simulink model "debugmotor"  (R2024a)
settings: Solver=VariableStepAuto  StartTime=0.0  StopTime=10  RelTol=1e-3
InitFcn:
  | stm32_pmsm_foc_data
undefined symbols (not defined in the file): PWM_frequency, target
libraries: mcbcontrolslib x7, simulink x2, slpidlib x2, mcbsensorlessestimatorlib x1, mcbplantlib x1, autolibpmsmexterior x1
settings Model: Creator=wsl  LastModifiedBy=wsl
settings DebuggingCC: ParameterPrecisionLossMsg=none

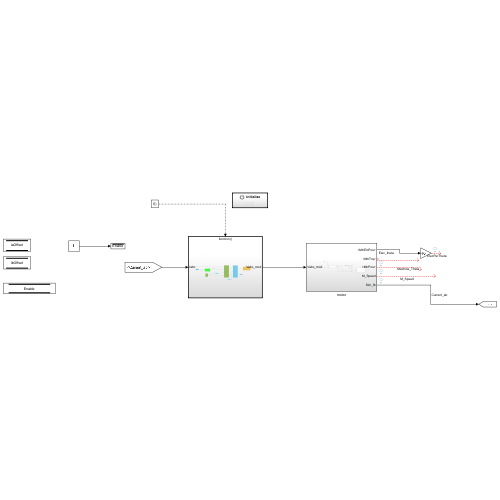
[thumbnail: Simulink's stored preview of the top-level diagram]
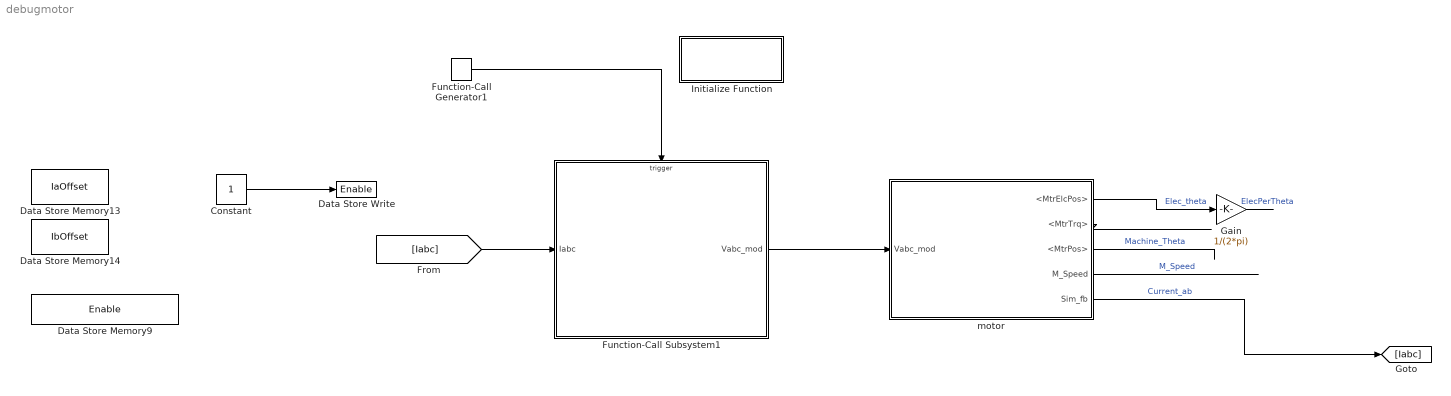
== system debugmotor ==
  Constant : Constant
  Data Store Memory13 : DataStoreMemory  DataStoreName=IaOffset  WriteAfterWriteMsg=warning  ShowAdditionalParam=off
  Data Store Memory14 : DataStoreMemory  DataStoreName=IbOffset  WriteAfterWriteMsg=warning  ShowAdditionalParam=off
  Data Store Memory9 : DataStoreMemory  DataStoreName=Enable  WriteAfterWriteMsg=warning  ShowAdditionalParam=off
  Data Store Write : DataStoreWrite  DataStoreName=Enable  IndexOptions=Index vector (dialog)  Indices=1  OutputSizes=1
  Function-Call Generator1 : simulink/Ports & Subsystems/Function-Call Generator  sample_time=Ts  numberOfIterations=1  DisallowWideOutput=off
  Function-Call Subsystem1 : Subsystem  TreatAsAtomicUnit=on
  Gain : Gain  Gain=1/(2*pi)
  Initialize Function : Subsystem  TreatAsAtomicUnit=on
  motor : Subsystem
  wires:
  motor/3(<MtrPos>) -> ?  "Machine_Theta"
  motor/5(Sim_fb) -> [Iabc]  "Current_ab"
  motor/2(<MtrTrq>) -> ?
  motor/4(M_Speed) -> ?  "M_Speed"
  Function-Call Generator1/1 -> Function-Call Subsystem1/Trigger
  Function-Call Subsystem1/1(Vabc_mod) -> motor/1(Vabc_mod)
  [Iabc] -> Function-Call Subsystem1/1(Iabc)
  Constant/1 -> Data Store Write/1
  motor/1(<MtrElcPos>) -> Gain/1  "Elec_theta"
  Gain/1 -> ?  "ElecPerTheta"

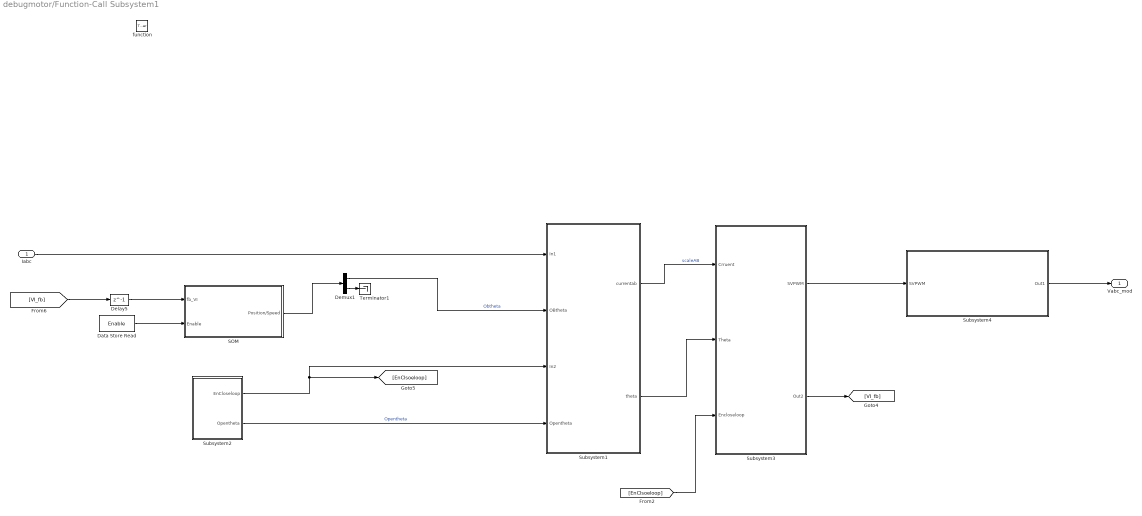
== system debugmotor/Function-Call Subsystem1 ==
  Iabc : Inport
  function : TriggerPort  TriggerType=function-call  VariantControl=(inherit)
  Data Store Read : DataStoreRead  DataStoreName=Enable  IndexOptions=Index vector (dialog)  Indices=1  OutputSizes=1
  Delay5 : Delay  DelayLength=1
  Demux1 : Demux  Outputs=2
  SOM : Subsystem
  Subsystem1 : Subsystem
  Subsystem2 : Subsystem
  Subsystem3 : Subsystem
  Subsystem4 : Subsystem
  Terminator1 : Terminator
  Vabc_mod : Outport
  wires:
  Subsystem1/1(currentab) -> Subsystem3/1(Crruent)  "scaleAB"
  Subsystem2/1(EnCloseloop) -> [EnClsoeloop], Subsystem1/3(In2)
  Subsystem2/2(Opentheta) -> Subsystem1/4(Opentheta)  "Opentheta"
  Demux1/2 -> Terminator1/1
  SOM/1(Position/Speed) -> Demux1/1
  Delay5/1 -> SOM/1(fb_VI)
  Data Store Read/1 -> SOM/2(Enable)
  [VI_fb] -> Delay5/1
  Demux1/1 -> Subsystem1/2(OBtheta)  "Obtheta"
  Iabc/1 -> Subsystem1/1(In1)
  Subsystem1/2(theta) -> Subsystem3/2(Theta)
  Subsystem3/2(Out2) -> [VI_fb]
  Subsystem3/1(SVPWM) -> Subsystem4/1(SVPWM)
  Subsystem4/1(Out1) -> Vabc_mod/1
  [EnClsoeloop] -> Subsystem3/3(Encloseloop)

== system debugmotor/Initialize Function ==
  Data Store Write : DataStoreWrite  DataStoreName=IaOffset  IndexOptions=Index vector (dialog)  Indices=1  OutputSizes=1
  Data Store Write1 : DataStoreWrite  DataStoreName=IbOffset  IndexOptions=Index vector (dialog)  Indices=1  OutputSizes=1
  Event Listener : EventListener  DisableCoverage=on  EventName=reset
  Testing get offset : Constant  Value=2075  OutDataTypeStr=int16
  Testing get offset1 : Constant  Value=2051  OutDataTypeStr=int16
  wires:
  Testing get offset1/1 -> Data Store Write/1
  Testing get offset/1 -> Data Store Write1/1

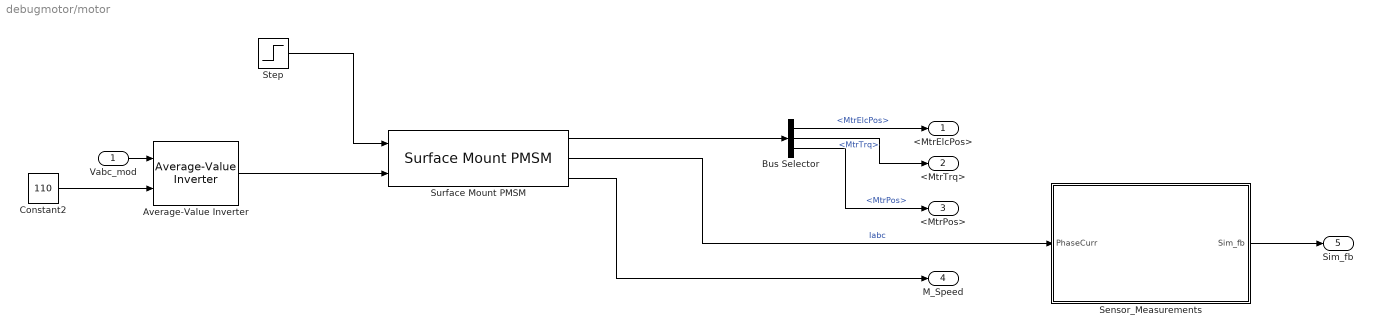
== system debugmotor/motor ==
  Vabc_mod : Inport
  Average-Value Inverter : mcbplantlib/Average-Value Inverter
  Bus Selector : BusSelector  OutputSignals=MtrElcPos,MtrTrq,MtrPos
  Constant2 : Constant  Value=110
  Sensor_Measurements : Subsystem
  Step : Step  After=0.15  SampleTime=0.01
  Surface Mount PMSM : autolibpmsmexterior/Surface Mount PMSM  port_config=Torque  sim_type=Discrete  Ts=5e-6  P=2  Rs=18.0  Ldq_=0.0407  KConstText=Back-emf constant (Ke):  lambda_pm=0.2205  Ke=29  Kt=1.323  mechanical=[0.0027, 4.924e-4, 0.05]  idq0=[0 0]  theta_init=0  omega_init=0  KConst=0.2205  lambda_pm_calc=0.079943  RefBlkName='autolibpmsmexterior/Surface Mount PMSM'  aMode=5  Ldq="[0.0017      0.0017]"
  <MtrElcPos> : Outport
  <MtrTrq> : Outport  Port=2
  <MtrPos> : Outport  Port=3
  M_Speed : Outport  Port=4
  Sim_fb : Outport  Port=5
  wires:
  Surface Mount PMSM/3 -> M_Speed/1
  Constant2/1 -> Average-Value Inverter/2
  Vabc_mod/1 -> Average-Value Inverter/1
  Average-Value Inverter/1 -> Surface Mount PMSM/2
  Step/1 -> Surface Mount PMSM/1
  Surface Mount PMSM/2 -> Sensor_Measurements/1(PhaseCurr)  "Iabc"
  Surface Mount PMSM/1 -> Bus Selector/1
  Bus Selector/1 -> <MtrElcPos>/1  "<MtrElcPos>"
  Bus Selector/2 -> <MtrTrq>/1  "<MtrTrq>"
  Bus Selector/3 -> <MtrPos>/1  "<MtrPos>"
  Sensor_Measurements/1(Sim_fb) -> Sim_fb/1

== system debugmotor/Function-Call Subsystem1/SOM ==
  fb_VI : Inport
  Enable : Inport  Port=2
  Demux1 : Demux
  Logical Operator : Logic  Operator=NOT  IconShape=distinctive  AllPortsSameDT=off  OutDataTypeStr=boolean
  Mux : Mux  Inputs=2
  Sliding Mode Observer : mcbsensorlessestimatorlib/Sliding Mode Observer  InputUnit=Per-unit  BlkSampleTime=50e-6  StatorResistance=18.1  StatorInductance=0.0407  MaxApplicationSpeed=2500  PolePairs=2  MaxStatorVoltage=110/1.732  MaxStatorCurrent=1  DisturbanceObserverGain=0.9  CurrentObserverGain=0.004938  CutoffFreq=500  PositionUnit=Per unit  PositionDataType=single  SpeedUnit=RPM  PerUnitSpeed=PU_System.N_base  SpeedDataType=single
  Position/Speed : Outport
  wires:
  Logical Operator/1 -> Sliding Mode Observer/5
  Mux/1 -> Position/Speed/1
  Demux1/3 -> Sliding Mode Observer/3  "Ialpha"
  fb_VI/1 -> Demux1/1
  Sliding Mode Observer/2 -> Mux/2
  Demux1/2 -> Sliding Mode Observer/2
  Sliding Mode Observer/1 -> Mux/1
  Enable/1 -> Logical Operator/1
  Demux1/1 -> Sliding Mode Observer/1
  Demux1/4 -> Sliding Mode Observer/4  "Ibeta"

== system debugmotor/Function-Call Subsystem1/Subsystem1 ==
  In1 : Inport
  OBtheta : Inport  Port=2
  In2 : Inport  Port=3
  Opentheta : Inport  Port=4
  Feedbackt_Current : Subsystem
  Switch : Switch  Criteria=u2 ~= 0  Threshold=0.1  SaturateOnIntegerOverflow=off  InputSameDT=off
  currentab : Outport
  theta : Outport  Port=2
  wires:
  Opentheta/1 -> Switch/3  "Eps"
  In2/1 -> Switch/2
  Switch/1 -> theta/1
  OBtheta/1 -> Switch/1
  In1/1 -> Feedbackt_Current/1(In1)
  Feedbackt_Current/1(currentab) -> currentab/1

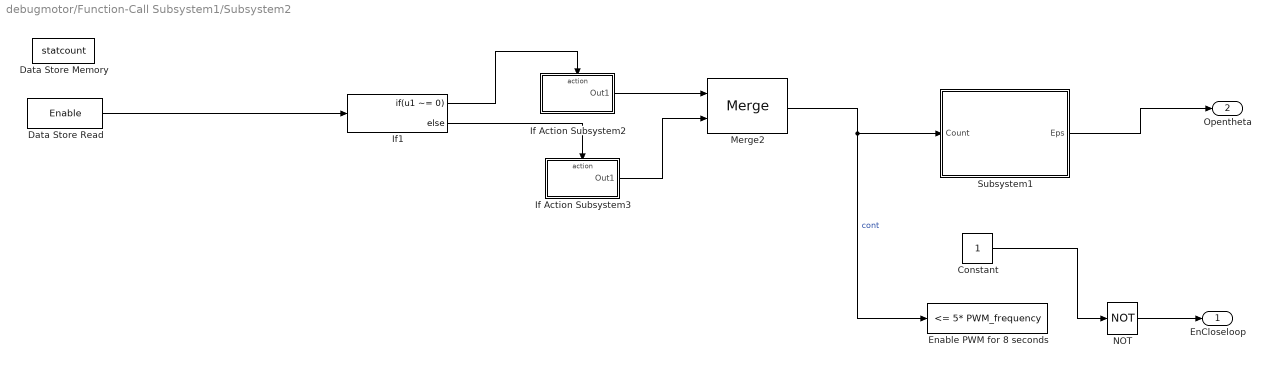
== system debugmotor/Function-Call Subsystem1/Subsystem2 ==
  Constant : Constant
  Data Store Memory : DataStoreMemory  DataStoreName=statcount  WriteAfterWriteMsg=warning  ShowAdditionalParam=off
  Data Store Read : DataStoreRead  DataStoreName=Enable  IndexOptions=Index vector (dialog)  Indices=1  OutputSizes=1
  Enable PWM for 8 seconds : simulink/Logic and Bit Operations/Compare To Constant  relop=<=  const=5* PWM_frequency  OutDataTypeStr=boolean
  If Action Subsystem2 : Subsystem  TreatAsAtomicUnit=on
  If Action Subsystem3 : Subsystem  TreatAsAtomicUnit=on
  If1 : If  IfExpression=u1 ~= 0
  Merge2 : Merge
  NOT : Logic  Operator=NOT  IconShape=distinctive  AllPortsSameDT=off  OutDataTypeStr=boolean
  Subsystem1 : Subsystem
  EnCloseloop : Outport  OutputWhenDisabled=reset  InitialOutput=0  VectorParamsAs1DForOutWhenUnconnected=off
  Opentheta : Outport  Port=2
  wires:
  If1/2 -> If Action Subsystem3/Action
  If1/1 -> If Action Subsystem2/Action
  If Action Subsystem3/1(Out1) -> Merge2/2
  If Action Subsystem2/1(Out1) -> Merge2/1
  Merge2/1 -> Enable PWM for 8 seconds/1, Subsystem1/1(Count)  "cont"
  Data Store Read/1 -> If1/1
  NOT/1 -> EnCloseloop/1
  Subsystem1/1(Eps) -> Opentheta/1
  Constant/1 -> NOT/1

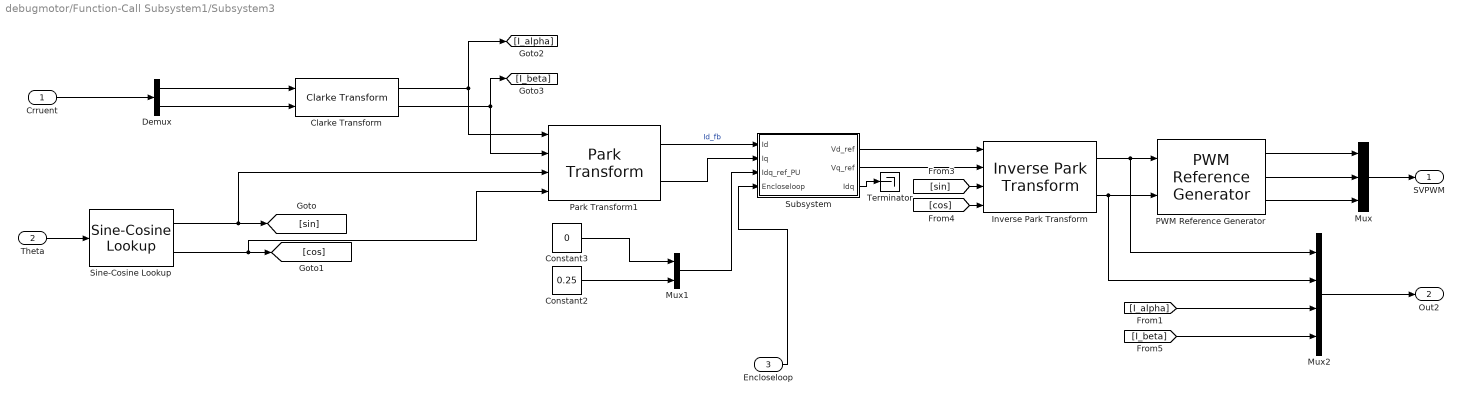
== system debugmotor/Function-Call Subsystem1/Subsystem3 ==
  Crruent : Inport
  Theta : Inport  Port=2
  Encloseloop : Inport  Port=3
  Clarke Transform : mcbcontrolslib/Clarke Transform  VariantControl=Variant2  PhaseInput=Two inputs  EnPowerInv=off
      settings: LibrarySourceBlock=mcbhdllib/Controls/Math Transforms/Clarke Transform
  Constant2 : Constant  Value=0.25  OutDataTypeStr=single
  Constant3 : Constant  Value=0  OutDataTypeStr=single
  Demux : Demux  Outputs=2
  Inverse Park Transform : mcbcontrolslib/Inverse Park Transform  PhaseInput=Two inputs  AxisAlignment=D-axis  ThetaInput=Sine and Cosine electrical position  AngleInput=Per-unit  N_points=1024
  Mux : Mux  Inputs=3
  Mux1 : Mux  Inputs=2
  Mux2 : Mux
  PWM Reference Generator : mcbcontrolslib/PWM Reference Generator  inSignal=Valphabeta  modType=SVM: space vector modulation
      settings: LibrarySourceBlock=mcblib/Controls/Math Transforms/PWM Reference Generator
  Park Transform1 : mcbcontrolslib/Park Transform  PhaseInput=Two inputs  AxisAlignment=D-axis  ThetaInput=Sine and Cosine electrical position  AngleInput=Per-unit  N_points=1024
      settings: LibrarySourceBlock=mcbhdllib/Controls/Math Transforms/Park Transform
  Sine-Cosine Lookup : mcbcontrolslib/Sine-Cosine Lookup  AngleInput=Per-unit  N_points=1024  DatatypeInput=Inherit from input  Datatype=single
  Subsystem : Subsystem
  Terminator : Terminator
  SVPWM : Outport
  Out2 : Outport  Port=2
  wires:
  Constant2/1 -> Mux1/2
  PWM Reference Generator/2 -> Mux/2
  Park Transform1/2 -> Subsystem/2(Iq)
  [cos] -> Inverse Park Transform/4
  Demux/2 -> Clarke Transform/2
  Sine-Cosine Lookup/1 -> Park Transform1/3, [sin]
  Subsystem/3(Idq) -> Terminator/1
  Demux/1 -> Clarke Transform/1
  Inverse Park Transform/1 -> Mux2/1, PWM Reference Generator/1
  Sine-Cosine Lookup/2 -> Park Transform1/4, [cos]
  Mux/1 -> SVPWM/1
  PWM Reference Generator/1 -> Mux/1
  Constant3/1 -> Mux1/1
  [sin] -> Inverse Park Transform/3
  Inverse Park Transform/2 -> Mux2/2, PWM Reference Generator/2
  [I_alpha] -> Mux2/3
  Clarke Transform/2 -> Park Transform1/2, [I_beta]
  Clarke Transform/1 -> Park Transform1/1, [I_alpha]
  Park Transform1/1 -> Subsystem/1(Id)  "Id_fb"
  [I_beta] -> Mux2/4
  Encloseloop/1 -> Subsystem/4(Encloseloop)
  Crruent/1 -> Demux/1
  PWM Reference Generator/3 -> Mux/3
  Subsystem/2(Vq_ref) -> Inverse Park Transform/2
  Mux1/1 -> Subsystem/3(Idq_ref_PU)
  Subsystem/1(Vd_ref) -> Inverse Park Transform/1
  Mux2/1 -> Out2/1
  Theta/1 -> Sine-Cosine Lookup/1

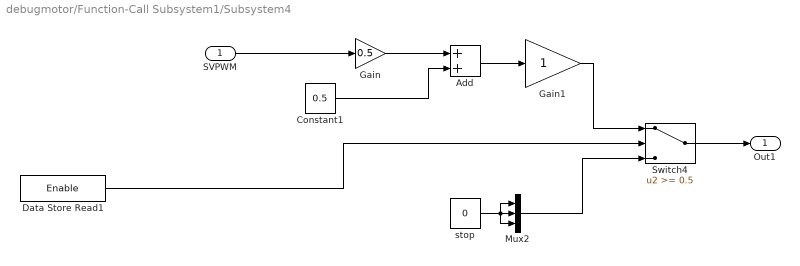
== system debugmotor/Function-Call Subsystem1/Subsystem4 ==
  SVPWM : Inport
  Add : Sum
  Constant1 : Constant  Value=0.5  OutDataTypeStr=single
  Data Store Read1 : DataStoreRead  DataStoreName=Enable  IndexOptions=Index vector (dialog)  Indices=1  OutputSizes=1
  Gain : Gain  Gain=0.5  OutDataTypeStr=single  RndMeth=Simplest
  Gain1 : Gain  OutDataTypeStr=single
  Mux2 : Mux  Inputs=3
  Switch4 : Switch  Threshold=0.5  SaturateOnIntegerOverflow=off  InputSameDT=off
  stop : Constant  Value=0  OutDataTypeStr=uint16
  Out1 : Outport
  wires:
  Gain1/1 -> Switch4/1
  Gain/1 -> Add/1
  Add/1 -> Gain1/1
  Data Store Read1/1 -> Switch4/2
  stop/1 -> Mux2/2, Mux2/3, Mux2/1
  Constant1/1 -> Add/2
  SVPWM/1 -> Gain/1
  Mux2/1 -> Switch4/3
  Switch4/1 -> Out1/1

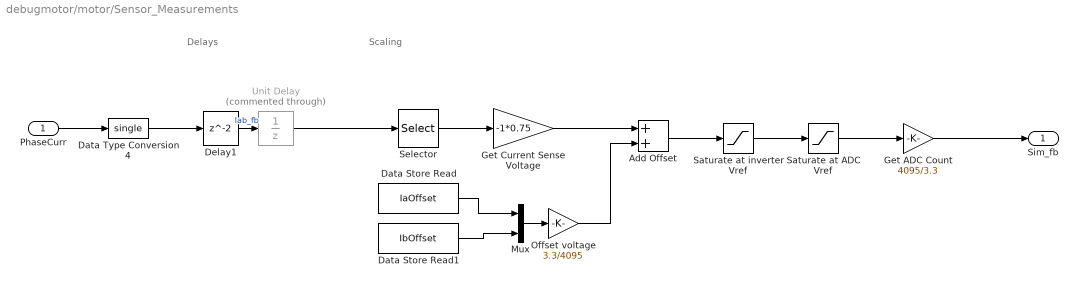
== system debugmotor/motor/Sensor_Measurements ==
  note: Scaling
  note: Delays
  PhaseCurr : Inport
  Add Offset : Sum  RndMeth=Simplest
  Data Store Read : DataStoreRead  DataStoreName=IaOffset  IndexOptions=Index vector (dialog)  Indices=1  OutputSizes=1
  Data Store Read1 : DataStoreRead  DataStoreName=IbOffset  IndexOptions=Index vector (dialog)  Indices=1  OutputSizes=1
  Data Type Conversion4 : DataTypeConversion  OutDataTypeStr=single  RndMeth=Simplest  SaturateOnIntegerOverflow=off
  Delay1 : Delay
  Get ADC Count : Gain  Gain=4095/3.3  OutMin=0  OutMax=target.ADC_MaxCount  OutDataTypeStr=uint16  RndMeth=Simplest
  Get Current Sense Voltage : Gain  Gain=-1*0.75  RndMeth=Simplest  OutDataTypeStr=Inherit: Same as input
  Mux : Mux  Inputs=2
  Offset voltage : Gain  Gain=3.3/4095  RndMeth=Simplest
  Saturate at ADC Vref : Saturate  UpperLimit=3.3  LowerLimit=0
  Saturate at inverter Vref : Saturate  UpperLimit=3.3  LowerLimit=0
  Selector : Selector  InputPortWidth=3  IndexOptions=Index vector (dialog)  Indices=[1 2]  OutputSizes=1
  Unit Delay : UnitDelay  Commented=through  SampleTime=-1  HasFrameUpgradeWarning=on
  Sim_fb : Outport  VectorParamsAs1DForOutWhenUnconnected=off
  wires:
  Delay1/1 -> Unit Delay/1  "Iab_fb"
  Data Type Conversion4/1 -> Delay1/1
  PhaseCurr/1 -> Data Type Conversion4/1
  Get ADC Count/1 -> Sim_fb/1
  Add Offset/1 -> Saturate at inverter Vref/1
  Saturate at inverter Vref/1 -> Saturate at ADC Vref/1
  Get Current Sense Voltage/1 -> Add Offset/1
  Saturate at ADC Vref/1 -> Get ADC Count/1
  Selector/1 -> Get Current Sense Voltage/1
  Offset voltage/1 -> Add Offset/2
  Unit Delay/1 -> Selector/1
  Data Store Read/1 -> Mux/1
  Data Store Read1/1 -> Mux/2
  Mux/1 -> Offset voltage/1

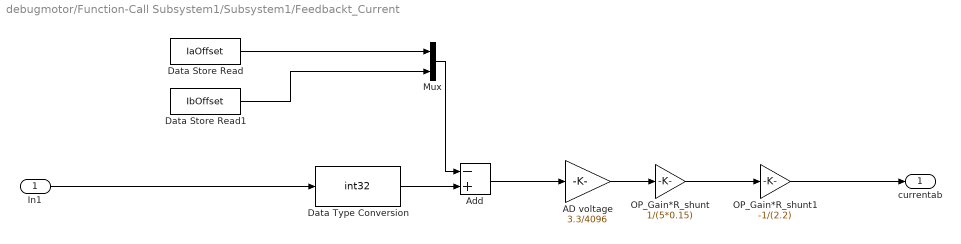
== system debugmotor/Function-Call Subsystem1/Subsystem1/Feedbackt_Current ==
  In1 : Inport
  AD voltage : Gain  Gain=3.3/4096  ParamDataTypeStr=single
  Add : Sum  Inputs=-+
  Data Store Read : DataStoreRead  DataStoreName=IaOffset  IndexOptions=Index vector (dialog)  Indices=1  OutputSizes=1
  Data Store Read1 : DataStoreRead  DataStoreName=IbOffset  IndexOptions=Index vector (dialog)  Indices=1  OutputSizes=1
  Data Type Conversion : DataTypeConversion  OutDataTypeStr=int32  ConvertRealWorld=Stored Integer (SI)  RndMeth=Simplest  SaturateOnIntegerOverflow=off
  Mux : Mux  Inputs=2
  OP_Gain*R_shunt : Gain  Gain=1/(5*0.15)  ParamDataTypeStr=single
  OP_Gain*R_shunt1 : Gain  Gain=-1/(2.2)  ParamDataTypeStr=single
  currentab : Outport
  wires:
  Add/1 -> AD voltage/1
  AD voltage/1 -> OP_Gain*R_shunt/1
  Mux/1 -> Add/1
  Data Type Conversion/1 -> Add/2
  Data Store Read/1 -> Mux/1
  Data Store Read1/1 -> Mux/2
  In1/1 -> Data Type Conversion/1
  OP_Gain*R_shunt1/1 -> currentab/1
  OP_Gain*R_shunt/1 -> OP_Gain*R_shunt1/1

== system debugmotor/Function-Call Subsystem1/Subsystem2/If Action Subsystem2 ==
  Action Port : ActionPort  ActionPortLabel=if(u1 ~= 0)
  Add1 : Sum  SaturateOnIntegerOverflow=on
  Constant : Constant  OutDataTypeStr=uint32
  Data Store Read : DataStoreRead  DataStoreName=statcount  IndexOptions=Index vector (dialog)  Indices=1  OutputSizes=1
  Data Store Write : DataStoreWrite  DataStoreName=statcount  IndexOptions=Index vector (dialog)  Indices=1  OutputSizes=1
  Out1 : Outport
  wires:
  Add1/1 -> Data Store Write/1, Out1/1
  Data Store Read/1 -> Add1/2
  Constant/1 -> Add1/1

== system debugmotor/Function-Call Subsystem1/Subsystem2/If Action Subsystem3 ==
  Action Port : ActionPort  ActionPortLabel=else
  Constant15 : Constant  Value=0  OutDataTypeStr=uint32
  Data Store Write : DataStoreWrite  DataStoreName=statcount  IndexOptions=Index vector (dialog)  Indices=1  OutputSizes=1
  Out1 : Outport
  wires:
  Constant15/1 -> Out1/1, Data Store Write/1

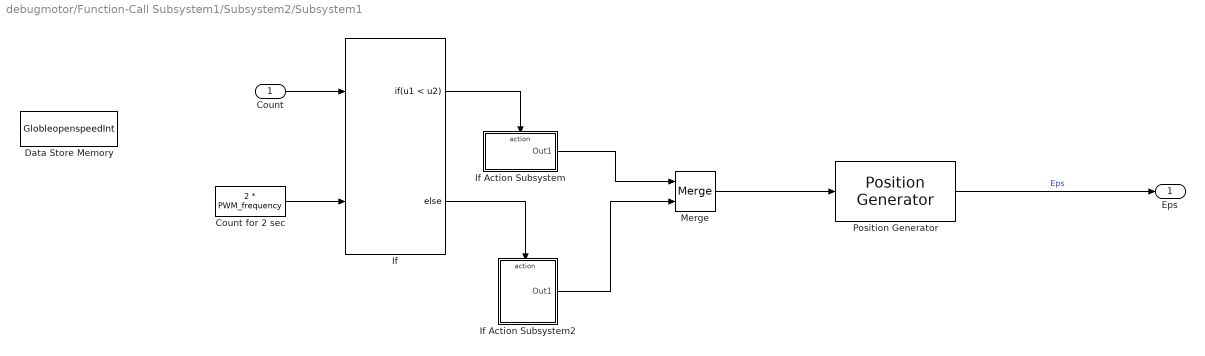
== system debugmotor/Function-Call Subsystem1/Subsystem2/Subsystem1 ==
  Count : Inport
  Count for 2 sec : Constant  Value=2 * PWM_frequency  OutDataTypeStr=uint32  SampleTime=-1
  Data Store Memory : DataStoreMemory  DataStoreName=GlobleopenspeedInt  WriteAfterWriteMsg=warning  ShowAdditionalParam=off
  If : If  NumInputs=2  IfExpression=u1 < u2
  If Action Subsystem : Subsystem  TreatAsAtomicUnit=on
  If Action Subsystem2 : Subsystem  TreatAsAtomicUnit=on
  Merge : Merge
  Position Generator : mcbcontrolslib/Position Generator  AngleOutput=Per-unit  ExternalReset=none  Offset=0
  Eps : Outport
  wires:
  If Action Subsystem/1(Out1) -> Merge/1
  If/1 -> If Action Subsystem/Action
  If Action Subsystem2/1(Out1) -> Merge/2
  Count/1 -> If/1
  If/2 -> If Action Subsystem2/Action
  Count for 2 sec/1 -> If/2
  Merge/1 -> Position Generator/1
  Position Generator/1 -> Eps/1  "Eps"

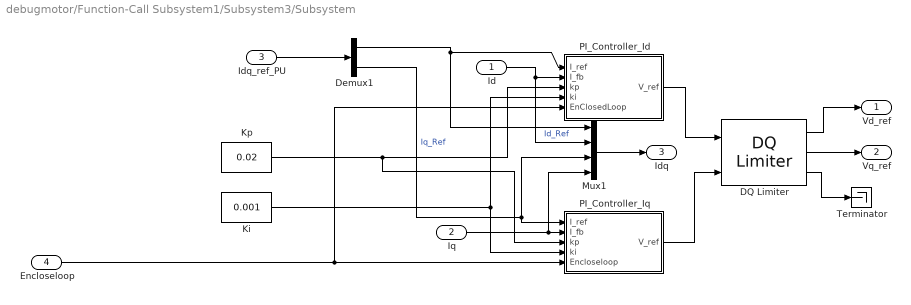
== system debugmotor/Function-Call Subsystem1/Subsystem3/Subsystem ==
  Id : Inport
  Iq : Inport  Port=2
  Idq_ref_PU : Inport  Port=3
  Encloseloop : Inport  Port=4
  DQ Limiter : mcbcontrolslib/DQ Limiter  satMethodInputType=Specify via dialog  satMethodSelected=D-Q equivalence  satLimitInputType=Specify via dialog  Vmax=0.95
  Demux1 : Demux  Outputs=2
  Ki : Constant  Value=0.001  OutDataTypeStr=single  SampleTime=-1
  Kp : Constant  Value=0.02  OutDataTypeStr=single  SampleTime=-1
  Mux1 : Mux
  PI_Controller_Id : Subsystem
  PI_Controller_Iq : Subsystem
  Terminator : Terminator
  Vd_ref : Outport  VectorParamsAs1DForOutWhenUnconnected=off
  Vq_ref : Outport  Port=2  VectorParamsAs1DForOutWhenUnconnected=off
  Idq : Outport  Port=3  VectorParamsAs1DForOutWhenUnconnected=off
  wires:
  DQ Limiter/1 -> Vd_ref/1
  Demux1/2 -> Mux1/3, PI_Controller_Iq/1(I_ref)  "Iq_Ref"
  Id/1 -> Mux1/2, PI_Controller_Id/2(I_fb)
  Demux1/1 -> Mux1/1, PI_Controller_Id/1(I_ref)  "Id_Ref"
  Idq_ref_PU/1 -> Demux1/1
  Iq/1 -> Mux1/4, PI_Controller_Iq/2(I_fb)
  Mux1/1 -> Idq/1
  PI_Controller_Iq/1(V_ref) -> DQ Limiter/2
  DQ Limiter/2 -> Vq_ref/1
  PI_Controller_Id/1(V_ref) -> DQ Limiter/1
  DQ Limiter/3 -> Terminator/1
  Kp/1 -> PI_Controller_Id/3(kp), PI_Controller_Iq/3(kp)
  Ki/1 -> PI_Controller_Iq/4(ki), PI_Controller_Id/4(ki)
  Encloseloop/1 -> PI_Controller_Id/5(EnClosedLoop), PI_Controller_Iq/5(Encloseloop)

== system debugmotor/Function-Call Subsystem1/Subsystem2/Subsystem1/If Action Subsystem ==
  Action Port : ActionPort  ActionPortLabel=if(u1 < u2)
  Constant : Constant  Value=0  OutDataTypeStr=single
  Data Store Write : DataStoreWrite  DataStoreName=GlobleopenspeedInt  IndexOptions=Index vector (dialog)  Indices=1  OutputSizes=1
  Out1 : Outport
  wires:
  Constant/1 -> Out1/1, Data Store Write/1

== system debugmotor/Function-Call Subsystem1/Subsystem2/Subsystem1/If Action Subsystem2 ==
  Action Port : ActionPort  ActionPortLabel=else
  Add1 : Sum
  Constant2 : Constant  Value=50e-6  VectorParams1D=off  OutDataTypeStr=single
  Data Store Read : DataStoreRead  DataStoreName=GlobleopenspeedInt  IndexOptions=Index vector (dialog)  Indices=1  OutputSizes=1
  Data Store Write : DataStoreWrite  DataStoreName=GlobleopenspeedInt  IndexOptions=Index vector (dialog)  Indices=1  OutputSizes=1
  Multiply1 : Gain  Gain=1/PWM_frequency  OutDataTypeStr=Inherit: Same as input
  Saturate to 'motor.calibSpeed' RPM : Saturate  UpperLimit=2 *300/60  LowerLimit=0
  Out1 : Outport
  wires:
  Constant2/1 -> Add1/1
  Saturate to 'motor.calibSpeed' RPM/1 -> Data Store Write/1, Multiply1/1
  Data Store Read/1 -> Add1/2
  Add1/1 -> Saturate to 'motor.calibSpeed' RPM/1
  Multiply1/1 -> Out1/1

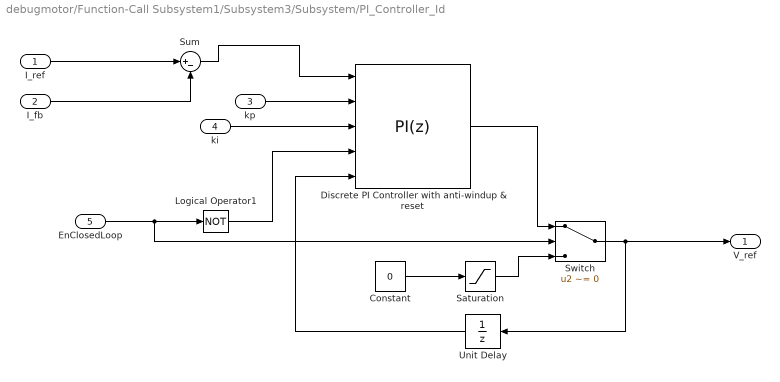
== system debugmotor/Function-Call Subsystem1/Subsystem3/Subsystem/PI_Controller_Id ==
  I_ref : Inport
  I_fb : Inport  Port=2
  kp : Inport  Port=3
  ki : Inport  Port=4
  EnClosedLoop : Inport  Port=5
  Constant : Constant  Value=0
  Discrete PI Controller with anti-windup & reset : slpidlib/PID Controller  Controller=PI  Form=Parallel  TimeDomain=Discrete-time  UseExternalTs=off  SampleTime=-1  IntegratorMethod=Forward Euler  FilterMethod=Forward Euler  ControllerParametersSource=external  P=1  I=1  UseKiTs=on  D=0  UseExternalDerivativeSource=off  N=100  UseFilter=on  TunerSelectOption=Transfer Function Based (PID Tuner App)  InitialConditionSource=external  InitialConditionForIntegrator=0  InitialConditionForFilter=0  DifferentiatorICPrevScaledInput=0  ExternalReset=level  TrackingMode=off  Kt=1  LimitOutput=on  SatLimitsSource=internal  UpperSaturationLimit=1  LowerSaturationLimit=-1  LinearizeAsGain=on  AntiWindupMode=clamping  Kb=1  LimitIntegrator=off  UpperIntegratorSaturationLimit=inf  LowerIntegratorSaturationLimit=-inf  RndMeth=Simplest  POutMin=[]  POutMax=[]  IOutMin=[]  IOutMax=[]  DOutMin=[]  DOutMax=[]  NOutMin=[]  NOutMax=[]  SumOutMin=[]  SumOutMax=[]  SaturationOutDataTypeStr=Inherit: Inherit via back propagation  SaturationOutMin=[]  SaturationOutMax=[]  PParamMin=[]  PParamMax=[]  IParamMin=[]  IParamMax=[]  DParamMin=[]  DParamMax=[]  NParamMin=[]  NParamMax=[]  KbParamMin=[]  KbParamMax=[]  KtParamMin=[]  KtParamMax=[]  KbOutMin=[]  KbOutMax=[]  KtOutMin=[]  KtOutMax=[]  IntegratorOutMin=[]  IntegratorOutMax=[]  FilterOutMin=[]  FilterOutMax=[]  SumI1OutMin=[]  SumI1OutMax=[]  SumI2OutMin=[]  SumI2OutMax=[]  SumI3OutMin=[]  SumI3OutMax=[]  SumI4OutMin=[]  SumI4OutMax=[]  SumDOutMin=[]  SumDOutMax=[]  DifferentiatorOutMin=[]  DifferentiatorOutMax=[]  FilterDiffOutCoefMin=[]  FilterDiffOutCoefMax=[]  ReciprocalOutMin=[]  ReciprocalOutMax=[]  SumDenOutMin=[]  SumDenOutMax=[]  SumNumOutMin=[]  SumNumOutMax=[]  DivideOutMin=[]  DivideOutMax=[]  UdiffTsProdOutMin=[]  UdiffTsProdOutMax=[]  NTsProdOutMin=[]  NTsProdOutMax=[]  UintegralTsProdOutMin=[]  UintegralTsProdOutMax=[]  UngainTsProdOutMin=[]  UngainTsProdOutMax=[]  ClampingZeroOutDataTypeStr=Inherit: Inherit via back propagation  ClampingZeroOutMin=[]  ClampingZeroOutMax=[]  FilterDenConstantOutDataTypeStr=Inherit: Inherit via back propagation  FilterDenConstantOutMin=[]  FilterDenConstantOutMax=[]  PCopyOutDataTypeStr=Inherit: Inherit via back propagation  PCopyOutMin=[]  PCopyOutMax=[]  NCopyOutDataTypeStr=Inherit: Inherit via back propagation  NCopyOutMin=[]  NCopyOutMax=[]  IntegratorContinuousStateAttributes=''  IntegratorStateMustResolveToSignalObject=off  IntegratorRTWStateStorageClass=Auto  FilterContinuousStateAttributes=''  FilterStateMustResolveToSignalObject=off  FilterRTWStateStorageClass=Auto  ParallelPVariant=ExternalParameters  IdealPVariant=Disabled  IVariant=ExternalParameters  DVariant=Disabled  IntegratorVariant=Discrete  SatVariant=Enabled  AWVariant=DiscClampingParallel  PCopyVariant=Disabled  TRVariant=Disabled  FdbkBlocksVariant=Forward  IdealPFdbkVariant=Disabled  SatFdbkVariant=Disabled  DerivativeFilterVariant=Disabled  NVariant=Disabled  NCopyVariant=Disabled_SignalSpec  FilterICVariant=Disabled  IntegratorICVariant=ExternalICs  ExternalResetVariant=ExternalReset  TRSumVariant=Passthrough  SumFdbkVariant=Disabled  SumVariant=Sum_PI  TsampFilterVariant=InternalTs  TsampNgainVariant=Passthrough  TsampIntegralVariant=Disabled_SignalSpec  ExternalSaturationOutDataTypeStr=Inherit: Same as second input  DerivativeSourceVariant=Disabled
      settings: LibrarySourceBlock=mcbcontrolslib/PI Controller
  Logical Operator1 : Logic  Operator=NOT  IconShape=distinctive  AllPortsSameDT=off  OutDataTypeStr=boolean
  Saturation : Saturate  LowerLimit=0.15  RndMeth=Simplest
  Sum : Sum  Inputs=|+-  OutDataTypeStr=Inherit: Same as first input
  Switch : Switch  Criteria=u2 ~= 0  RndMeth=Simplest  SaturateOnIntegerOverflow=off  InputSameDT=off
  Unit Delay : UnitDelay  SampleTime=-1  HasFrameUpgradeWarning=on
  V_ref : Outport  VectorParamsAs1DForOutWhenUnconnected=off
  wires:
  I_ref/1 -> Sum/1
  I_fb/1 -> Sum/2
  Sum/1 -> Discrete PI Controller with anti-windup & reset/1
  Logical Operator1/1 -> Discrete PI Controller with anti-windup & reset/4
  kp/1 -> Discrete PI Controller with anti-windup & reset/2
  ki/1 -> Discrete PI Controller with anti-windup & reset/3
  Saturation/1 -> Switch/3
  EnClosedLoop/1 -> Logical Operator1/1, Switch/2
  Unit Delay/1 -> Discrete PI Controller with anti-windup & reset/5
  Discrete PI Controller with anti-windup & reset/1 -> Switch/1
  Constant/1 -> Saturation/1
  Switch/1 -> V_ref/1, Unit Delay/1

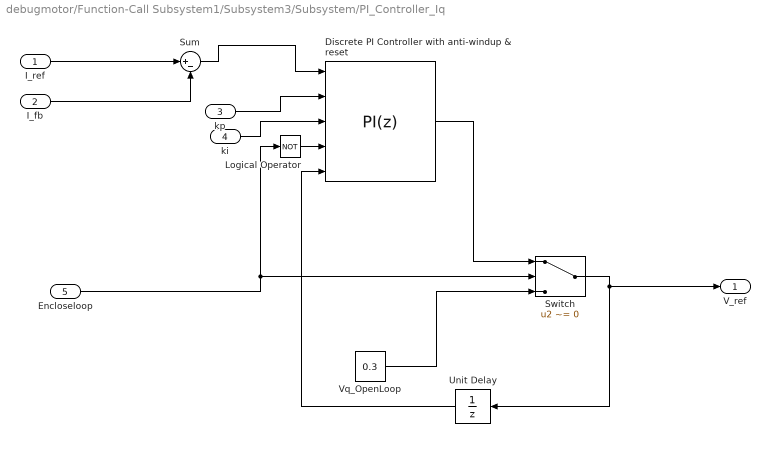
== system debugmotor/Function-Call Subsystem1/Subsystem3/Subsystem/PI_Controller_Iq ==
  I_ref : Inport
  I_fb : Inport  Port=2
  kp : Inport  Port=3
  ki : Inport  Port=4
  Encloseloop : Inport  Port=5
  Discrete PI Controller with anti-windup & reset : slpidlib/PID Controller  Controller=PI  Form=Parallel  TimeDomain=Discrete-time  UseExternalTs=off  SampleTime=-1  IntegratorMethod=Forward Euler  FilterMethod=Forward Euler  ControllerParametersSource=external  P=1  I=1  UseKiTs=on  D=0  UseExternalDerivativeSource=off  N=100  UseFilter=on  TunerSelectOption=Transfer Function Based (PID Tuner App)  InitialConditionSource=external  InitialConditionForIntegrator=0  InitialConditionForFilter=0  DifferentiatorICPrevScaledInput=0  ExternalReset=level  TrackingMode=off  Kt=1  LimitOutput=on  SatLimitsSource=internal  UpperSaturationLimit=1  LowerSaturationLimit=-1  LinearizeAsGain=on  AntiWindupMode=clamping  Kb=1  LimitIntegrator=off  UpperIntegratorSaturationLimit=inf  LowerIntegratorSaturationLimit=-inf  RndMeth=Simplest  POutMin=[]  POutMax=[]  IOutMin=[]  IOutMax=[]  DOutMin=[]  DOutMax=[]  NOutMin=[]  NOutMax=[]  SumOutMin=[]  SumOutMax=[]  SaturationOutDataTypeStr=Inherit: Inherit via back propagation  SaturationOutMin=[]  SaturationOutMax=[]  PParamMin=[]  PParamMax=[]  IParamMin=[]  IParamMax=[]  DParamMin=[]  DParamMax=[]  NParamMin=[]  NParamMax=[]  KbParamMin=[]  KbParamMax=[]  KtParamMin=[]  KtParamMax=[]  KbOutMin=[]  KbOutMax=[]  KtOutMin=[]  KtOutMax=[]  IntegratorOutMin=[]  IntegratorOutMax=[]  FilterOutMin=[]  FilterOutMax=[]  SumI1OutMin=[]  SumI1OutMax=[]  SumI2OutMin=[]  SumI2OutMax=[]  SumI3OutMin=[]  SumI3OutMax=[]  SumI4OutMin=[]  SumI4OutMax=[]  SumDOutMin=[]  SumDOutMax=[]  DifferentiatorOutMin=[]  DifferentiatorOutMax=[]  FilterDiffOutCoefMin=[]  FilterDiffOutCoefMax=[]  ReciprocalOutMin=[]  ReciprocalOutMax=[]  SumDenOutMin=[]  SumDenOutMax=[]  SumNumOutMin=[]  SumNumOutMax=[]  DivideOutMin=[]  DivideOutMax=[]  UdiffTsProdOutMin=[]  UdiffTsProdOutMax=[]  NTsProdOutMin=[]  NTsProdOutMax=[]  UintegralTsProdOutMin=[]  UintegralTsProdOutMax=[]  UngainTsProdOutMin=[]  UngainTsProdOutMax=[]  ClampingZeroOutDataTypeStr=Inherit: Inherit via back propagation  ClampingZeroOutMin=[]  ClampingZeroOutMax=[]  FilterDenConstantOutDataTypeStr=Inherit: Inherit via back propagation  FilterDenConstantOutMin=[]  FilterDenConstantOutMax=[]  PCopyOutDataTypeStr=Inherit: Inherit via back propagation  PCopyOutMin=[]  PCopyOutMax=[]  NCopyOutDataTypeStr=Inherit: Inherit via back propagation  NCopyOutMin=[]  NCopyOutMax=[]  IntegratorContinuousStateAttributes=''  IntegratorStateMustResolveToSignalObject=off  IntegratorRTWStateStorageClass=Auto  FilterContinuousStateAttributes=''  FilterStateMustResolveToSignalObject=off  FilterRTWStateStorageClass=Auto  ParallelPVariant=ExternalParameters  IdealPVariant=Disabled  IVariant=ExternalParameters  DVariant=Disabled  IntegratorVariant=Discrete  SatVariant=Enabled  AWVariant=DiscClampingParallel  PCopyVariant=Disabled  TRVariant=Disabled  FdbkBlocksVariant=Forward  IdealPFdbkVariant=Disabled  SatFdbkVariant=Disabled  DerivativeFilterVariant=Disabled  NVariant=Disabled  NCopyVariant=Disabled_SignalSpec  FilterICVariant=Disabled  IntegratorICVariant=ExternalICs  ExternalResetVariant=ExternalReset  TRSumVariant=Passthrough  SumFdbkVariant=Disabled  SumVariant=Sum_PI  TsampFilterVariant=InternalTs  TsampNgainVariant=Passthrough  TsampIntegralVariant=Disabled_SignalSpec  ExternalSaturationOutDataTypeStr=Inherit: Same as second input  DerivativeSourceVariant=Disabled
      settings: LibrarySourceBlock=mcbcontrolslib/PI Controller
  Logical Operator : Logic  Operator=NOT  IconShape=distinctive  AllPortsSameDT=off  OutDataTypeStr=boolean
  Sum : Sum  Inputs=|+-  OutDataTypeStr=Inherit: Same as first input
  Switch : Switch  Criteria=u2 ~= 0  RndMeth=Simplest  SaturateOnIntegerOverflow=off  InputSameDT=off
  Unit Delay : UnitDelay  SampleTime=-1  HasFrameUpgradeWarning=on
  Vq_OpenLoop : Constant  Value=0.3  OutDataTypeStr=single  SampleTime=-1
  V_ref : Outport  VectorParamsAs1DForOutWhenUnconnected=off
  wires:
  Encloseloop/1 -> Logical Operator/1, Switch/2
  I_fb/1 -> Sum/2
  I_ref/1 -> Sum/1
  Sum/1 -> Discrete PI Controller with anti-windup & reset/1
  Logical Operator/1 -> Discrete PI Controller with anti-windup & reset/4
  Switch/1 -> V_ref/1, Unit Delay/1
  kp/1 -> Discrete PI Controller with anti-windup & reset/2
  ki/1 -> Discrete PI Controller with anti-windup & reset/3
  Vq_OpenLoop/1 -> Switch/3
  Discrete PI Controller with anti-windup & reset/1 -> Switch/1
  Unit Delay/1 -> Discrete PI Controller with anti-windup & reset/5
